simulink model "Echo_cancel"  (R2019a)
settings: Solver=FixedStepDiscrete  StartTime=0.0  StopTime=10.0  RelTol=1e-3
libraries: dspadpt3 x1
settings Model: Creator=CIT_007  LastModifiedBy=CIT_007
settings OptimizationCC: DefaultParameterBehavior=Inlined  UseDivisionForNetSlopeComputation=on  GainParamInheritBuiltInType=on  UseFloatMulNetSlope=on  UseSpecifiedMinMax=on  InlineInvariantSignals=on  PassReuseOutputArgsAs=Individual arguments  ZeroExternalMemoryAtStartup=off  ZeroInternalMemoryAtStartup=off  NoFixptDivByZeroProtection=on  EfficientFloat2IntCast=on  LifeSpan=1  OptimizeBlockOrder=speed  DifferentSizesBufferReuse=on
settings DebuggingCC: ParameterTunabilityLossMsg=error
settings HardwareCC: ProdBitPerPointer=32  ProdBitPerSizeT=32  ProdBitPerPtrDiffT=32  ProdLargestAtomicInteger=Long  ProdLargestAtomicFloat=Double  ProdWordSize=32  ProdLongLongMode=on  ProdHWDeviceType=ARM Compatible->ARM Cortex
settings ModelReferenceCC: UpdateModelReferenceTargets=Force
settings SFSimCC: MATLABDynamicMemAlloc=off
settings RTWCC: SystemTargetFile=ert.tlc  TemplateMakefile=ert_default_tmf  GenerateReport=on  BuildConfiguration=Faster Runs  IncludeHyperlinkInReport=on  LaunchReport=on  GenerateTraceInfo=on  GenerateTraceReport=on  GenerateTraceReportSl=on  GenerateTraceReportSf=on  GenerateTraceReportEml=on  GenerateCodeMetricsReport=on
settings CodeAppCC: ForceParamTrailComments=on  IgnoreCustomStorageClasses=off  OperatorAnnotations=on  SimulinkDataObjDesc=on  SFDataObjDesc=on  CustomSymbolStrGlobalVar=rt$N$MeC  CustomSymbolStrType=$N$MeC  CustomSymbolStrField=$N$MeC  CustomSymbolStrFcn=$N$M$FeC  CustomSymbolStrFcnArg=rt$I$N$MeC  CustomSymbolStrBlkIO=rtb_$N$MeC  CustomSymbolStrTmpVar=$N$MeC  CustomSymbolStrMacro=$N$MeC  InsertBlockDesc=on  InternalIdentifier=Classic
settings ERTTargetCC: TargetLangStandard=C99 (ISO)  GenerateSampleERTMain=on  IncludeMdlTerminateFcn=off  CombineSignalStateStructs=on  SupportAbsoluteTime=off  SupportComplex=off  SupportNonInlinedSFcns=on  InlinedParameterPlacement=NonHierarchical  ERTCustomFileTemplate=example_file_process.tlc  ERTFilePackagingFormat=CompactWithDataFile

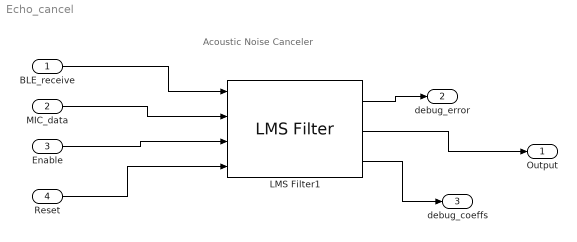
== system Echo_cancel ==
  note: Acoustic Noise Canceler
  BLE_receive : Inport  OutDataTypeStr=single
  MIC_data : Inport  Port=2  OutDataTypeStr=single
  Enable : Inport  Port=3  OutDataTypeStr=boolean
  Reset : Inport  Port=4  OutDataTypeStr=boolean
  LMS Filter1 : dspadpt3/LMS Filter  Algo=Normalized LMS  L=3  stepflag=Dialog  mu=0.02  leakage=1.0  ic=0  Adapt=on  resetflag=Non-zero sample  weights=on  addnparflag=off  roundingMode=Round  overflowMode=on  secondCoeffMode=Binary point scaling  secondCoeffWordLength=2  secondCoeffFracLength=15  prodOutput2Mode=Binary point scaling  prodOutput2FracLength=20  prodOutput3Mode=Binary point scaling  prodOutput3FracLength=20  prodOutput4Mode=Binary point scaling  prodOutput4FracLength=20  quotientMode=Binary point scaling  quotientFracLength=20  accum2Mode=Binary point scaling  accum2FracLength=20
      settings: SourceProductName=DSP System Toolbox  SourceProductBaseCode=DS  LockScale=on
  Output : Outport  OutDataTypeStr=single
  debug_error : Outport  Port=2  OutDataTypeStr=single
  debug_coeffs : Outport  Port=3  OutDataTypeStr=single
  wires:
  BLE_receive/1 -> LMS Filter1/1
  LMS Filter1/1 -> debug_error/1
  MIC_data/1 -> LMS Filter1/2
  LMS Filter1/2 -> Output/1
  Reset/1 -> LMS Filter1/4
  Enable/1 -> LMS Filter1/3
  LMS Filter1/3 -> debug_coeffs/1
